simulink model "Kalman_Filter"  (R2023b)
settings: Solver=VariableStepAuto  StartTime=0.0  StopTime=60  RelTol=1e-3
values from neighbouring files (symbols this model uses):
  Bw0 = [10;-20;-30]*pi/180    [main.m]
  Bwhat0 = [0;0;0]    [main.m]
  dt_gyros = 0.01    [main.m]
  dt_sim = 0.001    [main.m]
  dt_v1 = 1    [main.m]
  dt_v2 = 10    [main.m]
  nb_seed = randi([0, 2^32], 3, 1)    [main.m]
  nv1_seed = randi([0, 2^32], 3, 1)    [main.m]
  nv2_seed = randi([0, 2^32], 3, 1)    [main.m]
  nw_seed = randi([0, 2^32], 3, 1)    [main.m]
  P0 = diag([sigmaangle, sigmaangle, sigmaangle, sigmaomega, sigmaomega, sigmaomega])    [main.m]
  qhat0_BI = A2q(Ahat0_BI)    [main.m]
  sigmab = 0.1*pi/180    (= 0.00174532925199)    [main.m]
  sigmav1 = 1*pi/180    (= 0.0174532925199)    [main.m]
  sigmav2 = 0.1*pi/180    (= 0.00174532925199)    [main.m]
  sigmaw = 1*pi/180    (= 0.0174532925199)    [main.m]
  v1_I = [1;0;0]    [main.m]
  v2_I = [0;1;0]    [main.m]
undefined symbols (not defined in the file or in its folder): md, ms, rcb_B, rlb_B, X, Y, Z
libraries: sm_lib x10, nesl_utility x4, simulink x3
settings Model: Creator=allan  LastModifiedBy=allan

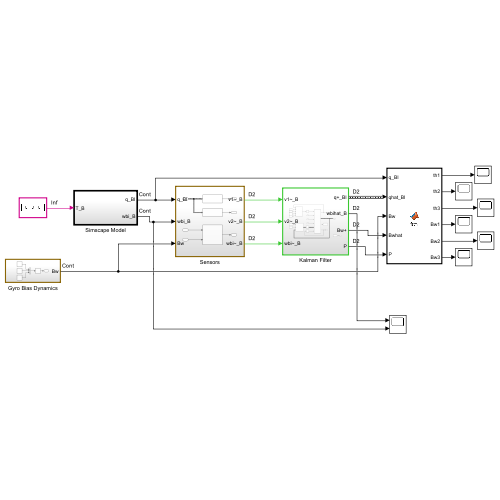
[thumbnail: Simulink's stored preview of the top-level diagram]
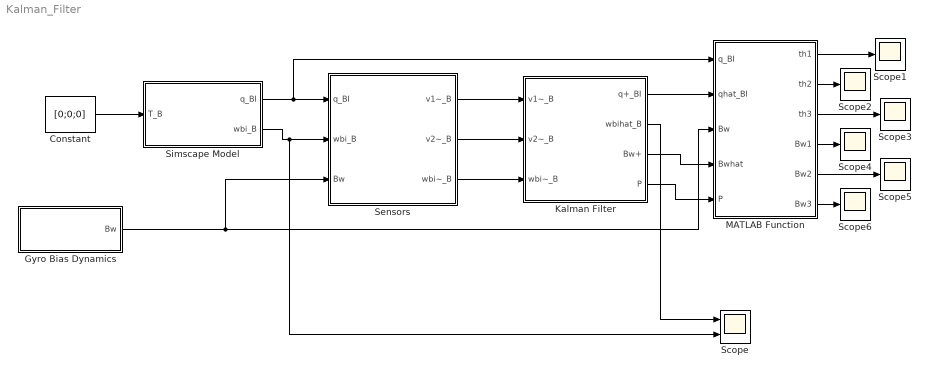
== system Kalman_Filter ==
  Constant : Constant  Value=[0;0;0]
  Gyro Bias Dynamics : Subsystem
  Kalman Filter : Subsystem
  MATLAB Function : MATLAB Function  TreatAsAtomicUnit=on
  Scope : Scope  NumInputPorts=2
  Scope{1..6} (6 alike) : Scope
  Sensors : Subsystem
  Simscape Model : Subsystem  TreatAsAtomicUnit=on
  wires:
  Constant/1 -> Simscape Model/1(T_B)
  Sensors/1(v1~_B) -> Kalman Filter/1(v1~_B)
  Sensors/2(v2~_B) -> Kalman Filter/2(v2~_B)
  Sensors/3(wbi~_B) -> Kalman Filter/3(wbi~_B)
  Kalman Filter/4(P) -> MATLAB Function/5(P)
  Kalman Filter/3(Bw+) -> MATLAB Function/4(Bwhat)
  Kalman Filter/2(wbihat_B) -> Scope/1
  Kalman Filter/1(q+_BI) -> MATLAB Function/2(qhat_BI)
  Simscape Model/1(q_BI) -> MATLAB Function/1(q_BI), Sensors/1(q_BI)
  Gyro Bias Dynamics/1(Bw) -> MATLAB Function/3(Bw), Sensors/3(Bw)
  Simscape Model/2(wbi_B) -> Scope/2, Sensors/2(wbi_B)
  MATLAB Function/1(th1) -> Scope1/1
  MATLAB Function/2(th2) -> Scope2/1
  MATLAB Function/3(th3) -> Scope3/1
  MATLAB Function/4(Bw1) -> Scope4/1
  MATLAB Function/5(Bw2) -> Scope5/1
  MATLAB Function/6(Bw3) -> Scope6/1

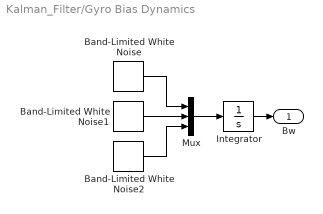
== system Kalman_Filter/Gyro Bias Dynamics ==
  Band-Limited White Noise : simulink/Sources/Band-Limited White Noise  Cov=[sigmab^2]  Ts=dt_sim  seed=[nb_seed(1)]
  Band-Limited White Noise1 : simulink/Sources/Band-Limited White Noise  Cov=[sigmab^2]  Ts=dt_sim  seed=[nb_seed(2)]
  Band-Limited White Noise2 : simulink/Sources/Band-Limited White Noise  Cov=[sigmab^2]  Ts=dt_sim  seed=[nb_seed(3)]
  Integrator : Integrator  InitialCondition=Bw0
  Mux : Mux  Inputs=3
  Bw : Outport
  wires:
  Integrator/1 -> Bw/1
  Mux/1 -> Integrator/1
  Band-Limited White Noise1/1 -> Mux/2
  Band-Limited White Noise/1 -> Mux/1
  Band-Limited White Noise2/1 -> Mux/3

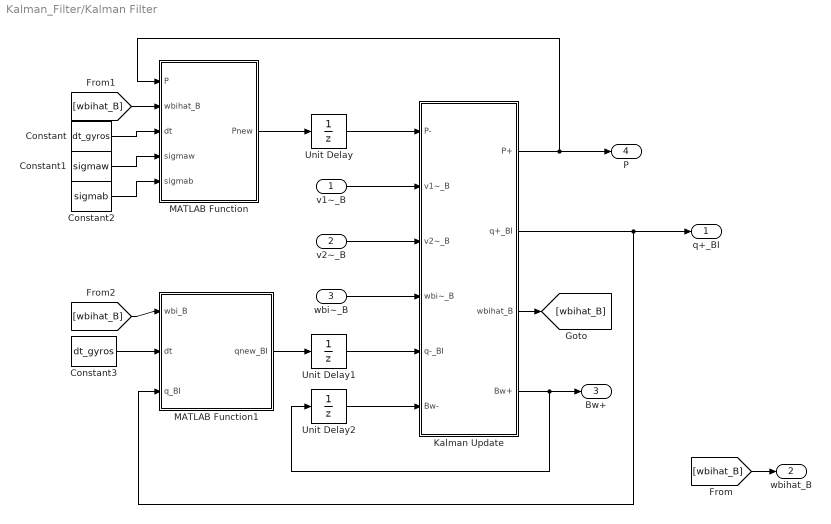
== system Kalman_Filter/Kalman Filter ==
  v1~_B : Inport
  v2~_B : Inport  Port=2
  wbi~_B : Inport  Port=3
  Constant : Constant  Value=dt_gyros
  Constant1 : Constant  Value=sigmaw
  Constant2 : Constant  Value=sigmab
  Constant3 : Constant  Value=dt_gyros
  Kalman Update : Subsystem
  MATLAB Function : MATLAB Function  TreatAsAtomicUnit=on
  MATLAB Function1 : MATLAB Function  TreatAsAtomicUnit=on
  Unit Delay : UnitDelay  InitialCondition=P0  SampleTime=-1  HasFrameUpgradeWarning=on
  Unit Delay1 : UnitDelay  InitialCondition=qhat0_BI  SampleTime=-1  HasFrameUpgradeWarning=on
  Unit Delay2 : UnitDelay  InitialCondition=Bwhat0  SampleTime=-1  HasFrameUpgradeWarning=on
  q+_BI : Outport
  wbihat_B : Outport  Port=2
  Bw+ : Outport  Port=3
  P : Outport  Port=4
  wires:
  Unit Delay/1 -> Kalman Update/1(P-)
  v1~_B/1 -> Kalman Update/2(v1~_B)
  v2~_B/1 -> Kalman Update/3(v2~_B)
  wbi~_B/1 -> Kalman Update/4(wbi~_B)
  Unit Delay1/1 -> Kalman Update/5(q-_BI)
  Unit Delay2/1 -> Kalman Update/6(Bw-)
  Kalman Update/1(P+) -> MATLAB Function/1(P), P/1
  Kalman Update/2(q+_BI) -> MATLAB Function1/3(q_BI), q+_BI/1
  Kalman Update/4(Bw+) -> Unit Delay2/1, Bw+/1
  [wbihat_B] -> wbihat_B/1
  Kalman Update/3(wbihat_B) -> [wbihat_B]
  MATLAB Function/1(Pnew) -> Unit Delay/1
  [wbihat_B] -> MATLAB Function/2(wbihat_B)
  MATLAB Function1/1(qnew_BI) -> Unit Delay1/1
  [wbihat_B] -> MATLAB Function1/1(wbi_B)
  Constant3/1 -> MATLAB Function1/2(dt)
  Constant/1 -> MATLAB Function/3(dt)
  Constant1/1 -> MATLAB Function/4(sigmaw)
  Constant2/1 -> MATLAB Function/5(sigmab)

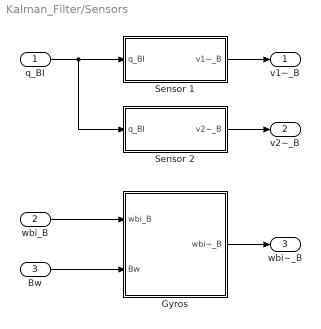
== system Kalman_Filter/Sensors ==
  q_BI : Inport
  wbi_B : Inport  Port=2
  Bw : Inport  Port=3
  Gyros : Subsystem
  Sensor 1 : Subsystem
  Sensor 2 : Subsystem
  v1~_B : Outport
  v2~_B : Outport  Port=2
  wbi~_B : Outport  Port=3
  wires:
  q_BI/1 -> Sensor 2/1(q_BI), Sensor 1/1(q_BI)
  Sensor 1/1(v1~_B) -> v1~_B/1
  Gyros/1(wbi~_B) -> wbi~_B/1
  wbi_B/1 -> Gyros/1(wbi_B)
  Bw/1 -> Gyros/2(Bw)
  Sensor 2/1(v2~_B) -> v2~_B/1

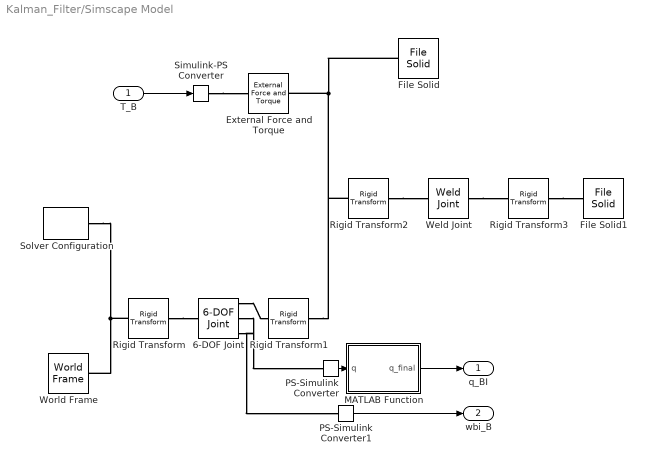
== system Kalman_Filter/Simscape Model ==
  T_B : Inport
  6-DOF Joint : sm_lib/Joints/6-DOF Joint  JointMode=Normal  SenseConstraintForce=off  SenseConstraintForceX=off  SenseConstraintForceY=off  SenseConstraintForceZ=off  SenseConstraintTorque=off  SenseConstraintTorqueX=off  SenseConstraintTorqueY=off  SenseConstraintTorqueZ=off  SenseTotalForce=off  SenseTotalForceX=off  SenseTotalForceY=off  SenseTotalForceZ=off  SenseTotalTorque=off  SenseTotalTorqueX=off  SenseTotalTorqueY=off  SenseTotalTorqueZ=off  CompositeWrenchDir=FollowerOnBase  CompositeWrenchFrame=BaseFrame  PxEquilibriumPosition=0  PxEquilibriumPositionUnits=m  PxSpringStiffness=0  PxSpringStiffnessUnits=N/m  PxDampingCoefficient=0  PxDampingCoefficientUnits=N/(m/s)  PxTorqueActuationMode=NoTorque  PxMotionActuationMode=ComputedMotion  PxSensePosition=off  PxSenseVelocity=off  PxSenseAcceleration=off  PxSenseTorqueForce=off  PxSenseLowerLimitTorqueForce=off  PxSenseUpperLimitTorqueForce=off  PxLowerLimitSpecify=off  PxLowerLimitBound=-1  PxLowerLimitBoundUnits=m  PxLowerLimitStiffness=1e6  PxLowerLimitStiffnessUnits=N/m  PxLowerLimitDamping=1e3  PxLowerLimitDampingUnits=N/(m/s)  PxLowerLimitTransitionRegionWidth=1e-4  PxLowerLimitTransitionRegionWidthUnits=m  PxUpperLimitSpecify=off  PxUpperLimitBound=1  PxUpperLimitBoundUnits=m  PxUpperLimitStiffness=1e6  PxUpperLimitStiffnessUnits=N/m  PxUpperLimitDamping=1e3  PxUpperLimitDampingUnits=N/(m/s)  PxUpperLimitTransitionRegionWidth=1e-4  PxUpperLimitTransitionRegionWidthUnits=m  PxPositionTargetSpecify=off  PxPositionTargetPriority=High  PxPositionTargetValue=0  PxPositionTargetValueUnits=m  PxVelocityTargetSpecify=off  PxVelocityTargetPriority=High  PxVelocityTargetValue=0  PxVelocityTargetValueUnits=m/s  PyEquilibriumPosition=0  PyEquilibriumPositionUnits=m  PySpringStiffness=0  PySpringStiffnessUnits=N/m  PyDampingCoefficient=0  PyDampingCoefficientUnits=N/(m/s)  PyTorqueActuationMode=NoTorque  PyMotionActuationMode=ComputedMotion  PySensePosition=off  PySenseVelocity=off  PySenseAcceleration=off  PySenseTorqueForce=off  PySenseLowerLimitTorqueForce=off  PySenseUpperLimitTorqueForce=off  PyLowerLimitSpecify=off  PyLowerLimitBound=-1  PyLowerLimitBoundUnits=m  PyLowerLimitStiffness=1e6  PyLowerLimitStiffnessUnits=N/m  PyLowerLimitDamping=1e3  PyLowerLimitDampingUnits=N/(m/s)  PyLowerLimitTransitionRegionWidth=1e-4  PyLowerLimitTransitionRegionWidthUnits=m  PyUpperLimitSpecify=off  PyUpperLimitBound=1  PyUpperLimitBoundUnits=m  PyUpperLimitStiffness=1e6  PyUpperLimitStiffnessUnits=N/m  PyUpperLimitDamping=1e3  PyUpperLimitDampingUnits=N/(m/s)  PyUpperLimitTransitionRegionWidth=1e-4  PyUpperLimitTransitionRegionWidthUnits=m  PyPositionTargetSpecify=off  PyPositionTargetPriority=High  PyPositionTargetValue=0  PyPositionTargetValueUnits=m  PyVelocityTargetSpecify=off  PyVelocityTargetPriority=High  PyVelocityTargetValue=0  PyVelocityTargetValueUnits=m/s  PzEquilibriumPosition=0  PzEquilibriumPositionUnits=m  PzSpringStiffness=0  PzSpringStiffnessUnits=N/m  PzDampingCoefficient=0  PzDampingCoefficientUnits=N/(m/s)  PzTorqueActuationMode=NoTorque  PzMotionActuationMode=ComputedMotion  PzSensePosition=off  PzSenseVelocity=off  PzSenseAcceleration=off  PzSenseTorqueForce=off  PzSenseLowerLimitTorqueForce=off  PzSenseUpperLimitTorqueForce=off  PzLowerLimitSpecify=off  PzLowerLimitBound=-1  PzLowerLimitBoundUnits=m  PzLowerLimitStiffness=1e6  PzLowerLimitStiffnessUnits=N/m  PzLowerLimitDamping=1e3  PzLowerLimitDampingUnits=N/(m/s)  PzLowerLimitTransitionRegionWidth=1e-4  PzLowerLimitTransitionRegionWidthUnits=m  PzUpperLimitSpecify=off  PzUpperLimitBound=1  PzUpperLimitBoundUnits=m  PzUpperLimitStiffness=1e6  PzUpperLimitStiffnessUnits=N/m  PzUpperLimitDamping=1e3  PzUpperLimitDampingUnits=N/(m/s)  PzUpperLimitTransitionRegionWidth=1e-4  PzUpperLimitTransitionRegionWidthUnits=m  PzPositionTargetSpecify=off  PzPositionTargetPriority=High  PzPositionTargetValue=0  PzPositionTargetValueUnits=m  PzVelocityTargetSpecify=off  PzVelocityTargetPriority=High  PzVelocityTargetValue=0  PzVelocityTargetValueUnits=m/s  SphEqPosRotationMethod=None  SphEqPosRotationAngleUnits=deg  SphEqPosRotationStandardAxis=+Z  SphEqPosRotationAngle=0.0  SphEqPosRotationArbitraryAxis=[0 0 1]  SphEqPosFollAlignAxisA=+X  SphEqPosBaseAlignAxisA=+Y  SphEqPosFollAlignAxisB=+Y  SphEqPosBaseAlignAxisB=+Z  SphEqPosRotationSequenceAxes=FollowerAxes  SphEqPosRotationSequence=XYX  SphEqPosRotationSequenceAngles=[0 0 0]  SphEqPosRotationSequenceAnglesUnits=deg  SphEqPosRotationMatrix=[1 0 0; 0 1 0; 0 0 1]  SphEqPosQuaternion=[1 0 0 0]  SphSpringStiffness=0  SphSpringStiffnessUnits=N*m/deg  SphDampingCoefficient=0  SphDampingCoefficientUnits=N*m/(deg/s)  SphActuateTorqueX=off  SphActuateTorqueY=off  SphActuateTorqueZ=off  SphActuateTorque=off  SphTorqueActuationMode=NoTorque  SphMotionActuationMode=ComputedMotion  SphActuationFrame=BaseFrame  SphSensePosition=on  SphSenseVelocityX=off  SphSenseVelocityY=off  SphSenseVelocityZ=off  SphSenseVelocity=on  SphSenseAccelerationX=off  SphSenseAccelerationY=off  SphSenseAccelerationZ=off  SphSenseAcceleration=off  SphSenseTorqueX=off  SphSenseTorqueY=off  SphSenseTorqueZ=off  SphSenseTorqueForce=off  SphSenseLowerLimitTorqueMag=off  SphSenseUpperLimitTorqueMag=off  SphSensingFrame=FollowerFrame  SphLowerLimitSpecify=off  SphLowerLimitBound=15  SphLowerLimitBoundUnits=deg  SphLowerLimitStiffness=1e4  SphLowerLimitStiffnessUnits=N*m/deg  SphLowerLimitDamping=10  SphLowerLimitDampingUnits=N*m/(deg/s)  SphLowerLimitTransitionRegionWidth=0.1  SphLowerLimitTransitionRegionWidthUnits=deg  SphUpperLimitSpecify=off  SphUpperLimitBound=45  SphUpperLimitBoundUnits=deg  SphUpperLimitStiffness=1e4  SphUpperLimitStiffnessUnits=N*m/deg  SphUpperLimitDamping=10  SphUpperLimitDampingUnits=N*m/(deg/s)  SphUpperLimitTransitionRegionWidth=0.1  SphUpperLimitTransitionRegionWidthUnits=deg  SphPositionTargetRotationMethod=RotationMatrix  SphPositionTargetRotationAngleUnits=deg  SphPositionTargetRotationStandardAxis=+Z  SphPositionTargetRotationAngle=0.0  SphPositionTargetRotationArbitraryAxis=[0 0 1]  SphPositionTargetFollAlignAxisA=+X  SphPositionTargetBaseAlignAxisA=+Y  SphPositionTargetFollAlignAxisB=+Y  SphPositionTargetBaseAlignAxisB=+Z  SphPositionTargetRotationSequenceAxes=FollowerAxes  SphPositionTargetRotationSequence=XYX  SphPositionTargetRotationSequenceAngles=[0 0 0]  SphPositionTargetRotationSequenceAnglesUnits=deg  SphPositionTargetRotationMatrix=A0_IB  SphPositionTargetQuaternion=[1 0 0 0]  SphPositionTargetSpecify=on  SphPositionTargetPriority=High  SphVelocityTargetValue=wbi0_B  SphVelocityTargetValueUnits=rad/s  SphVelocityTargetSpecify=on  SphVelocityTargetPriority=High  SphVelocityTargetInFollowerFrame=on
  External Force and Torque : sm_lib/Forces and Torques/External Force and Torque  ForceResolutionFrame=AttachedFrame  EnableForceX=off  EnableForceY=off  EnableForceZ=off  EnableForce=off  TorqueResolutionFrame=AttachedFrame  EnableTorqueX=off  EnableTorqueY=off  EnableTorqueZ=off  EnableTorque=on
  File Solid : sm_lib/Body Elements/File Solid  ExtGeomFileName=D:\Spacecraft Attitude Control Theory\Attitude Dynamics\Structure.STL  UnitType=Custom  ExtGeomFileUnits=mm  StepReaderType=HEX  ExportConvexHullGeometry=off  InertiaType=Custom  Mass=ms  MassUnits=kg  CenterOfMass=rsb_B  CenterOfMassUnits=m  MomentsOfInertia=Ms_S_B  MomentsOfInertiaUnits=kg*m^2  ProductsOfInertia=Ps_S_B  ProductsOfInertiaUnits=kg*m^2  BasedOnType=DensityFromFile  Density=1000  DensityUnits=kg/m^3  DoExposeReferenceFrame=on  SerializedFrames=<Frames/>  GraphicType=FromGeometry  MarkerShape=Sphere  MarkerSize=10  GraphicVisPropType=SimpleVisualProperties  GraphicDiffuseColor=[1.0 0.0 0.0]  GraphicSpecularColor=[0.5 0.5 0.5 1.0]  GraphicAmbientColor=[0.15 0.15 0.15 1.0]  GraphicEmissiveColor=[0.0 0.0 0.0 1.0]  GraphicShininess=75  GraphicOpacity=1.0
  File Solid1 : sm_lib/Body Elements/File Solid  ExtGeomFileName=D:\Spacecraft Attitude Control Theory\Attitude Dynamics\Deployable.STL  UnitType=Custom  ExtGeomFileUnits=mm  StepReaderType=HEX  ExportConvexHullGeometry=off  InertiaType=Custom  Mass=md  MassUnits=kg  CenterOfMass=rdb_B  CenterOfMassUnits=m  MomentsOfInertia=Md_D_B  MomentsOfInertiaUnits=kg*m^2  ProductsOfInertia=Pd_D_B  ProductsOfInertiaUnits=kg*m^2  BasedOnType=DensityFromFile  Density=1000  DensityUnits=kg/m^3  DoExposeReferenceFrame=on  SerializedFrames=<Frames/>  GraphicType=FromGeometry  MarkerShape=Sphere  MarkerSize=10  GraphicVisPropType=SimpleVisualProperties  GraphicDiffuseColor=[0.5 0.5 0.5]  GraphicSpecularColor=[0.5 0.5 0.5 1.0]  GraphicAmbientColor=[0.15 0.15 0.15 1.0]  GraphicEmissiveColor=[0.0 0.0 0.0 1.0]  GraphicShininess=75  GraphicOpacity=1.0
  MATLAB Function : MATLAB Function  TreatAsAtomicUnit=on
  PS-Simulink Converter : nesl_utility/PS-Simulink Converter  PhysicalDomain=network_engine_domain  SubClassName=ps_output  LeftPortType=input  RightPortType=output  PseudoPeriodic=off  Frequencies=[]  VectorFormat=inherit  Unit=inherit  AffineConversion=off
  PS-Simulink Converter1 : nesl_utility/PS-Simulink Converter  PhysicalDomain=network_engine_domain  SubClassName=ps_output  LeftPortType=input  RightPortType=output  PseudoPeriodic=off  Frequencies=[]  VectorFormat=inherit  Unit=inherit  AffineConversion=off
  Rigid Transform : sm_lib/Frames and Transforms/Rigid Transform  TranslationMethod=Cartesian  TranslationStandardOffset=0  TranslationStandardOffsetUnits=m  TranslationStandardAxis=+Z  TranslationCartesianOffset=rcb_B  TranslationCartesianOffsetUnits=m  TranslationROffset=0  TranslationROffsetUnits=m  TranslationZOffset=0  TranslationZOffsetUnits=m  TranslationThetaOffset=0  TranslationThetaOffsetUnits=deg  RotationMethod=None  RotationAngleUnits=deg  RotationStandardAxis=+Z  RotationAngle=0.0  RotationArbitraryAxis=[0 0 1]  FollAlignAxisA=+X  BaseAlignAxisA=+Y  FollAlignAxisB=+Y  BaseAlignAxisB=+Z  RotationSequenceAxes=FollowerAxes  RotationSequence=XYX  RotationSequenceAngles=[0 0 0]  RotationSequenceAnglesUnits=deg  RotationMatrix=[1 0 0; 0 1 0; 0 0 1]  Quaternion=[1 0 0 0]
  Rigid Transform1 : sm_lib/Frames and Transforms/Rigid Transform  TranslationMethod=Cartesian  TranslationStandardOffset=0  TranslationStandardOffsetUnits=m  TranslationStandardAxis=+Z  TranslationCartesianOffset=-rcb_B  TranslationCartesianOffsetUnits=m  TranslationROffset=0  TranslationROffsetUnits=m  TranslationZOffset=0  TranslationZOffsetUnits=m  TranslationThetaOffset=0  TranslationThetaOffsetUnits=deg  RotationMethod=None  RotationAngleUnits=deg  RotationStandardAxis=+Z  RotationAngle=0.0  RotationArbitraryAxis=[0 0 1]  FollAlignAxisA=+X  BaseAlignAxisA=+Y  FollAlignAxisB=+Y  BaseAlignAxisB=+Z  RotationSequenceAxes=FollowerAxes  RotationSequence=XYX  RotationSequenceAngles=[0 0 0]  RotationSequenceAnglesUnits=deg  RotationMatrix=[1 0 0; 0 1 0; 0 0 1]  Quaternion=[1 0 0 0]
  Rigid Transform2 : sm_lib/Frames and Transforms/Rigid Transform  TranslationMethod=Cartesian  TranslationStandardOffset=0  TranslationStandardOffsetUnits=m  TranslationStandardAxis=+Z  TranslationCartesianOffset=rlb_B  TranslationCartesianOffsetUnits=m  TranslationROffset=0  TranslationROffsetUnits=m  TranslationZOffset=0  TranslationZOffsetUnits=m  TranslationThetaOffset=0  TranslationThetaOffsetUnits=deg  RotationMethod=None  RotationAngleUnits=deg  RotationStandardAxis=+Z  RotationAngle=0.0  RotationArbitraryAxis=[0 0 1]  FollAlignAxisA=+X  BaseAlignAxisA=+Y  FollAlignAxisB=+Y  BaseAlignAxisB=+Z  RotationSequenceAxes=FollowerAxes  RotationSequence=XYX  RotationSequenceAngles=[0 0 0]  RotationSequenceAnglesUnits=deg  RotationMatrix=[1 0 0; 0 1 0; 0 0 1]  Quaternion=[1 0 0 0]
  Rigid Transform3 : sm_lib/Frames and Transforms/Rigid Transform  TranslationMethod=Cartesian  TranslationStandardOffset=0  TranslationStandardOffsetUnits=m  TranslationStandardAxis=+Z  TranslationCartesianOffset=-rlb_B  TranslationCartesianOffsetUnits=m  TranslationROffset=0  TranslationROffsetUnits=m  TranslationZOffset=0  TranslationZOffsetUnits=m  TranslationThetaOffset=0  TranslationThetaOffsetUnits=deg  RotationMethod=None  RotationAngleUnits=deg  RotationStandardAxis=+Z  RotationAngle=0.0  RotationArbitraryAxis=[0 0 1]  FollAlignAxisA=+X  BaseAlignAxisA=+Y  FollAlignAxisB=+Y  BaseAlignAxisB=+Z  RotationSequenceAxes=FollowerAxes  RotationSequence=XYX  RotationSequenceAngles=[0 0 0]  RotationSequenceAnglesUnits=deg  RotationMatrix=[1 0 0; 0 1 0; 0 0 1]  Quaternion=[1 0 0 0]
  Simulink-PS Converter : nesl_utility/Simulink-PS Converter  PhysicalDomain=network_engine_domain  SubClassName=ps_input  LeftPortType=input  RightPortType=output  PseudoPeriodic=off  Frequencies=[]  NoiseDistribution=none  NoiseParameters=[]  Unit=1  AffineConversion=off  FilteringAndDerivatives=provide  SimscapeFilterOrder=1  InputFilterTimeConstant=0.001  UdotUserProvided=0
  Solver Configuration : nesl_utility/Solver Configuration  PhysicalDomain=network_engine_domain  SubClassName=solver  LeftPortType=input  RightPortType=generic  Tones=[]  Harmonics=[]  SimulateNoise=off  Profile=off  UseLocalSampling=off  EnableSwitchedLinearOptims=on  FrequencyDomain=off  UseCCode=off  RelTol=0.001  AbsTol=0.001  MinStep=1e-09  ToWorkspace=off  RevertToSquareIcSolve=off  NumHomotopyIterations=100  PhasorMode=off  PhasorModeNumHarmonics=1  ConsistencySolver=NEWTON_XTOL_AFTER_FTOL  IndexReductionMethod=DerivativeReplacement  DoDC=off  ResidualTolerance=1e-09  ConsistencyTolSource=GLOBAL  ConsistencyAbsTol=0.001  ConsistencyRelTol=0.001  ConsistencyTolFactor=0.1  UseLocalSolver=off  LocalSolverChoice=NE_BACKWARD_EULER_ADVANCER  ResolveIndetEquations=on  FunctionEvalNumThread=1  LocalSolverSampleTime=0.001  DoFixedCost=off  MaxNonlinIter=3  MaxModeIter=2  ComputeImpulses=off  ImpulseIterations=2  LinearAlgebra=auto  LinearAlgebraNumThread=0  EquationFormulation=NE_TIME_EF  DelaysMemoryBudget=1024  AutomaticFiltering=on  FilteringTimeConstant=0.001  PartitionStorageMethod=AS_NEEDED  PartitionMemoryBudget=1024  PartitionMethod=ROBUST  MultibodyUseLocalSolver=off  MultibodyLocalSolverChoice=ODE1  MultibodyLocalSolverSampleTime=0.001
  Weld Joint : sm_lib/Joints/Weld Joint  JointMode=Normal  SenseConstraintForce=off  SenseConstraintForceX=off  SenseConstraintForceY=off  SenseConstraintForceZ=off  SenseConstraintTorque=off  SenseConstraintTorqueX=off  SenseConstraintTorqueY=off  SenseConstraintTorqueZ=off  SenseTotalForce=off  SenseTotalForceX=off  SenseTotalForceY=off  SenseTotalForceZ=off  SenseTotalTorque=off  SenseTotalTorqueX=off  SenseTotalTorqueY=off  SenseTotalTorqueZ=off  CompositeWrenchDir=FollowerOnBase  CompositeWrenchFrame=BaseFrame
  World Frame : sm_lib/Frames and Transforms/World Frame
  q_BI : Outport  OutDataTypeStr=Bus: qBus  VectorParamsAs1DForOutWhenUnconnected=off
  wbi_B : Outport  Port=2  VectorParamsAs1DForOutWhenUnconnected=off
  wires:
  T_B/1 -> Simulink-PS Converter/1
  PS-Simulink Converter1/1 -> wbi_B/1
  PS-Simulink Converter/1 -> MATLAB Function/1(q)
  MATLAB Function/1(q_final) -> q_BI/1
  connections:
  Solver Configuration/RConn1 -- Rigid Transform/LConn1 -- World Frame/RConn1
  Rigid Transform/RConn1 -- 6-DOF Joint/LConn1
  6-DOF Joint/RConn1 -- Rigid Transform1/LConn1
  Simulink-PS Converter/RConn1 -- External Force and Torque/LConn1
  Rigid Transform3/RConn1 -- File Solid1/RConn1
  Weld Joint/RConn1 -- Rigid Transform3/LConn1
  Rigid Transform2/RConn1 -- Weld Joint/LConn1
  File Solid/RConn1 -- External Force and Torque/RConn1 -- Rigid Transform1/RConn1 -- Rigid Transform2/LConn1
  6-DOF Joint/RConn2 -- PS-Simulink Converter/LConn1
  6-DOF Joint/RConn3 -- PS-Simulink Converter1/LConn1

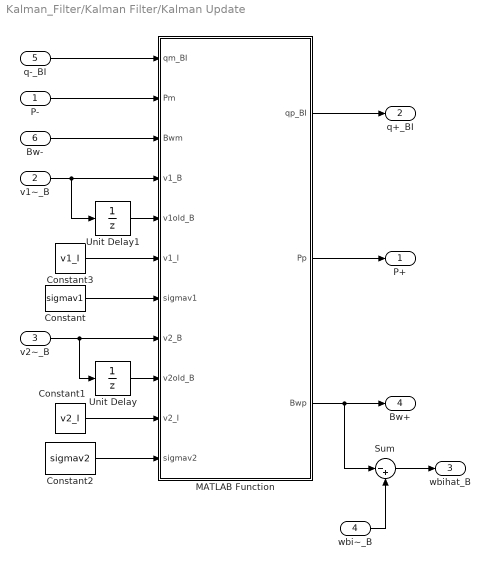
== system Kalman_Filter/Kalman Filter/Kalman Update ==
  P- : Inport
  v1~_B : Inport  Port=2
  v2~_B : Inport  Port=3
  wbi~_B : Inport  Port=4
  q-_BI : Inport  Port=5  OutDataTypeStr=Bus: qBus
  Bw- : Inport  Port=6
  Constant : Constant  Value=sigmav1
  Constant1 : Constant  Value=v2_I
  Constant2 : Constant  Value=sigmav2
  Constant3 : Constant  Value=v1_I
  MATLAB Function : MATLAB Function  TreatAsAtomicUnit=on
  Sum : Sum  Inputs=|-+
  Unit Delay : UnitDelay  SampleTime=-1  HasFrameUpgradeWarning=on
  Unit Delay1 : UnitDelay  SampleTime=-1  HasFrameUpgradeWarning=on
  P+ : Outport
  q+_BI : Outport  Port=2  OutDataTypeStr=Bus: qBus
  wbihat_B : Outport  Port=3
  Bw+ : Outport  Port=4
  wires:
  MATLAB Function/1(qp_BI) -> q+_BI/1
  MATLAB Function/2(Pp) -> P+/1
  MATLAB Function/3(Bwp) -> Sum/1, Bw+/1
  Sum/1 -> wbihat_B/1
  wbi~_B/1 -> Sum/2
  Constant2/1 -> MATLAB Function/11(sigmav2)
  Constant1/1 -> MATLAB Function/10(v2_I)
  v2~_B/1 -> Unit Delay/1, MATLAB Function/8(v2_B)
  Unit Delay/1 -> MATLAB Function/9(v2old_B)
  Constant/1 -> MATLAB Function/7(sigmav1)
  Constant3/1 -> MATLAB Function/6(v1_I)
  v1~_B/1 -> Unit Delay1/1, MATLAB Function/4(v1_B)
  Unit Delay1/1 -> MATLAB Function/5(v1old_B)
  P-/1 -> MATLAB Function/2(Pm)
  Bw-/1 -> MATLAB Function/3(Bwm)
  q-_BI/1 -> MATLAB Function/1(qm_BI)

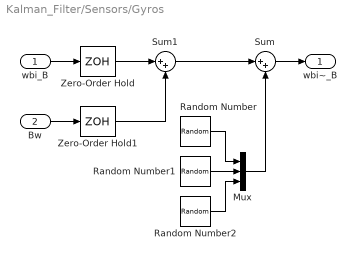
== system Kalman_Filter/Sensors/Gyros ==
  wbi_B : Inport
  Bw : Inport  Port=2
  Mux : Mux  Inputs=3
  Random Number : RandomNumber  Variance=sigmaw^2  Seed=nw_seed(1)  SampleTime=dt_gyros
  Random Number1 : RandomNumber  Variance=sigmaw^2  Seed=nw_seed(2)  SampleTime=dt_gyros
  Random Number2 : RandomNumber  Variance=sigmaw^2  Seed=nw_seed(3)  SampleTime=dt_gyros
  Sum : Sum  Inputs=|++
  Sum1 : Sum  Inputs=|++
  Zero-Order Hold : ZeroOrderHold  SampleTime=dt_gyros
  Zero-Order Hold1 : ZeroOrderHold  SampleTime=dt_gyros
  wbi~_B : Outport
  wires:
  wbi_B/1 -> Zero-Order Hold/1
  Bw/1 -> Zero-Order Hold1/1
  Zero-Order Hold/1 -> Sum1/1
  Zero-Order Hold1/1 -> Sum1/2
  Sum1/1 -> Sum/1
  Mux/1 -> Sum/2
  Sum/1 -> wbi~_B/1
  Random Number1/1 -> Mux/2
  Random Number2/1 -> Mux/3
  Random Number/1 -> Mux/1

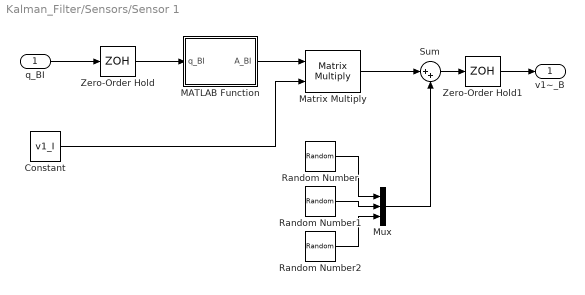
== system Kalman_Filter/Sensors/Sensor 1 ==
  q_BI : Inport  OutDataTypeStr=Bus: qBus
  Constant : Constant  Value=v1_I  SampleTime=dt_v1
  MATLAB Function : MATLAB Function  TreatAsAtomicUnit=on
  Matrix Multiply : Product  Multiplication=Matrix(*)
  Mux : Mux  Inputs=3
  Random Number : RandomNumber  Variance=sigmav1^2  Seed=nv1_seed(1)  SampleTime=dt_v1
  Random Number1 : RandomNumber  Variance=sigmav1^2  Seed=nv1_seed(2)  SampleTime=dt_v1
  Random Number2 : RandomNumber  Variance=sigmav1^2  Seed=nv1_seed(3)  SampleTime=dt_v1
  Sum : Sum  Inputs=|++
  Zero-Order Hold : ZeroOrderHold  SampleTime=dt_v1
  Zero-Order Hold1 : ZeroOrderHold  SampleTime=dt_gyros
  v1~_B : Outport
  wires:
  q_BI/1 -> Zero-Order Hold/1
  Zero-Order Hold/1 -> MATLAB Function/1(q_BI)
  MATLAB Function/1(A_BI) -> Matrix Multiply/1
  Constant/1 -> Matrix Multiply/2
  Matrix Multiply/1 -> Sum/1
  Mux/1 -> Sum/2
  Random Number1/1 -> Mux/2
  Random Number/1 -> Mux/1
  Random Number2/1 -> Mux/3
  Sum/1 -> Zero-Order Hold1/1
  Zero-Order Hold1/1 -> v1~_B/1

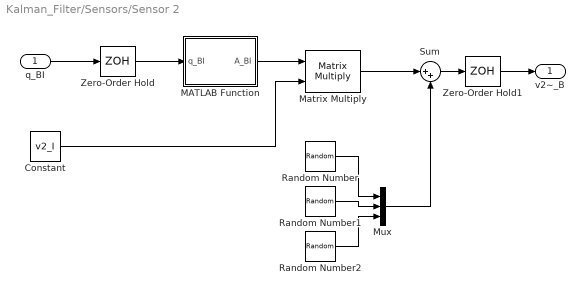
== system Kalman_Filter/Sensors/Sensor 2 ==
  q_BI : Inport  OutDataTypeStr=Bus: qBus
  Constant : Constant  Value=v2_I  SampleTime=dt_v2
  MATLAB Function : MATLAB Function  TreatAsAtomicUnit=on
  Matrix Multiply : Product  Multiplication=Matrix(*)
  Mux : Mux  Inputs=3
  Random Number : RandomNumber  Variance=sigmav2^2  Seed=nv2_seed(1)  SampleTime=dt_v2
  Random Number1 : RandomNumber  Variance=sigmav2^2  Seed=nv2_seed(2)  SampleTime=dt_v2
  Random Number2 : RandomNumber  Variance=sigmav2^2  Seed=nv2_seed(3)  SampleTime=dt_v2
  Sum : Sum  Inputs=|++
  Zero-Order Hold : ZeroOrderHold  SampleTime=dt_v2
  Zero-Order Hold1 : ZeroOrderHold  SampleTime=dt_gyros
  v2~_B : Outport
  wires:
  q_BI/1 -> Zero-Order Hold/1
  Zero-Order Hold/1 -> MATLAB Function/1(q_BI)
  MATLAB Function/1(A_BI) -> Matrix Multiply/1
  Constant/1 -> Matrix Multiply/2
  Matrix Multiply/1 -> Sum/1
  Mux/1 -> Sum/2
  Random Number1/1 -> Mux/2
  Random Number/1 -> Mux/1
  Random Number2/1 -> Mux/3
  Sum/1 -> Zero-Order Hold1/1
  Zero-Order Hold1/1 -> v2~_B/1

== matlab function Kalman_Filter/Simscape Model/MATLAB Function ==
  data: q input; q_final output Bus: qBus
function q_final = fcn(q)

q_final.s = q(1);
q_final.v = q(2:4);

== matlab function Kalman_Filter/Sensors/Sensor 1/MATLAB Function ==
  data: q_BI input Bus: qBus; A_BI output
function A_BI = fcn(q_BI)

A_BI = q2A(q_BI);

== matlab function Kalman_Filter/Sensors/Sensor 2/MATLAB Function ==
  data: q_BI input Bus: qBus; A_BI output
function A_BI = fcn(q_BI)

A_BI = q2A(q_BI);

== matlab function Kalman_Filter/Kalman Filter/MATLAB Function ==
  data: P input; Pnew output; wbihat_B input; dt input; sigmaw input; sigmab input
function Pnew = fcn(P, wbihat_B, dt, sigmaw, sigmab)

wX = X(wbihat_B);

wmag = norm(wbihat_B);

I3 = eye(3);
O3 = zeros(3,3);

Phi11 = I3 - wX*sin(wmag*dt)/wmag + wX*wX*(1-cos(wmag*dt))/wmag^2;
Phi12 = wX*(1-cos(wmag*dt))/wmag^2 - I3*dt - wX*wX*(wmag*dt - sin(wmag*dt))/wmag^3;

Phi = [Phi11,Phi12; O3, I3];

Qd = [(sigmaw^2*dt + 1/3*sigmab^2*dt^3)*I3, -(1/2*sigmab^2*dt^2)*I3;
    -(1/2*sigmab^2*dt^2)*I3, (sigmab^2*dt)*I3];

Pnew = Phi*P*Phi' + Qd;

Pnew = (Pnew + Pnew')/2;

== matlab function Kalman_Filter/Kalman Filter/MATLAB Function1 ==
  data: wbi_B input; qnew_BI output Bus: qBus; dt input; q_BI input Bus: qBus
function qnew_BI = fcn(wbi_B, dt, q_BI)

w_mag = norm(wbi_B);

psi = sin(1/2*w_mag*dt)*wbi_B/w_mag;

psiX = X(psi);

qnew_BI.s = cos(1/2*w_mag*dt)*q_BI.s - psi'*q_BI.v;
qnew_BI.v = psi*q_BI.s + (cos(1/2*w_mag*dt)*eye(3) - psiX)*q_BI.v;

qnew_BI = qUnit(qnew_BI);

== matlab function Kalman_Filter/Kalman Filter/Kalman Update/MATLAB Function ==
  data: qm_BI input Bus: qBus; qp_BI output Bus: qBus; Pm input; Bwm input; v1_B input; v1old_B input; v1_I input; sigmav1 input; v2_B input; v2old_B input; v2_I input; sigmav2 input; Pp output; Bwp output
function [qp_BI, Pp, Bwp] = fcn(qm_BI, Pm, Bwm, v1_B, v1old_B, v1_I, ...
    sigmav1, v2_B, v2old_B, v2_I, sigmav2)

if v1_B ~= v1old_B

    [qp_BI, Pp, Bwp] = update(qm_BI, Pm, Bwm, v1_B, v1_I, sigmav1);

else

    qp_BI = qm_BI;
    Pp = Pm;
    Bwp = Bwm;

end

if v2_B ~= v2old_B

    [qp_BI, Pp, Bwp] = update(qp_BI, Pp, Bwp, v2_B, v2_I, sigmav2);

end

end

function [qp_BI, Pp, Bwp] = update(qm_BI, Pm, Bwm, v_B, v_I, sigmav)

    Ahat_BI = q2A(qm_BI);

    vhat_B = Ahat_BI*v_I;

    vhat_BX = X(vhat_B);

    H = [vhat_BX, zeros(3,3)];

    R = sigmav^2*eye(3);

    K = Pm*H'/(H*Pm*H' + R);
    
    dx = K*(v_B - vhat_B);

    dth = dx(1:3);

    dBw = dx(4:6);

    qp_BI.s = qm_BI.s - 1/2*(qm_BI.v')*dth;
    qp_BI.v = qm_BI.v + 1/2*(qm_BI.s*eye(3) + X(qm_BI.v))*dth;

    qp_BI = qUnit(qp_BI);

    Pp = (eye(6) - K*H)*Pm;
    Pp = (Pp + Pp')/2;
    Bwp = Bwm + dBw;

end

== matlab function Kalman_Filter/MATLAB Function ==
  data: q_BI input Bus: qBus; th1 output; qhat_BI input Bus: qBus; Bw input; Bwhat input; P input; th2 output; th3 output; Bw1 output; Bw2 output; Bw3 output
function [th1, th2, th3, Bw1, Bw2, Bw3] = fcn(q_BI, qhat_BI, Bw, Bwhat, P)

[axis, angle] = q2e(q_BI);
th = angle*axis;

[axis, angle] = q2e(qhat_BI);
thhat = angle*axis;

th1 = [th(1); thhat(1); thhat(1) + 3*sqrt(P(1,1)); thhat(1) - 3*sqrt(P(1,1))];
th2 = [th(2); thhat(2); thhat(2) + 3*sqrt(P(2,2)); thhat(2) - 3*sqrt(P(2,2))];
th3 = [th(3); thhat(3); thhat(3) + 3*sqrt(P(3,3)); thhat(3) - 3*sqrt(P(3,3))];

Bw1 = [Bw(1); Bwhat(1); Bwhat(1)+3*sqrt(P(4,4)); Bwhat(1) - 3*sqrt(P(4,4))];
Bw2 = [Bw(2); Bwhat(2); Bwhat(2)+3*sqrt(P(5,5)); Bwhat(2) - 3*sqrt(P(5,5))];
Bw3 = [Bw(3); Bwhat(3); Bwhat(3)+3*sqrt(P(6,6)); Bwhat(3) - 3*sqrt(P(6,6))];
